simulink library "TempSensor"  (Simulink 7.6)
settings: Solver=ode1  StartTime=0.0  StopTime=Inf  FixedStep=0.001  RelTol=1e-3
PostLoadFcn:
  | , if any(exist('dsrtsu_mdlpostloadfcn', 'file') == [2, 3, 6]), try dsrtsu_mdlpostloadfcn('Execute', bdroot); catch fprintf('Error in PostLoadFcn (dsrtsu_mdlpostloadfcn) for model "%s":\n %s\n', bdroot, lasterr); end, end,
libraries: rti1401lib_dac_type1 x1
settings Model: DSRTSU_INTERNAL_RTI_VER=370  DSRTSU_INTERNAL_RTI_TYPE=rti1401  Creator=ses  LastModifiedBy=ses

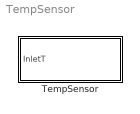
== system TempSensor ==
  TempSensor : Subsystem  mask{R0=200, TSnsrVect=[1 3.8285e-3 -5.85e-7], PuUpR=1000, PuUpU=5, CalBias=-0.006}
      mask prompts: R0 "Nominal Resistance [Ohm]"; TSnsrVect "Sensor Characteristic Vector"; PuUpR "Pull-up Resistance [Ohm]"; PuUpU "Pull-up Voltage [V]"; CalBias "Calibration Bias"

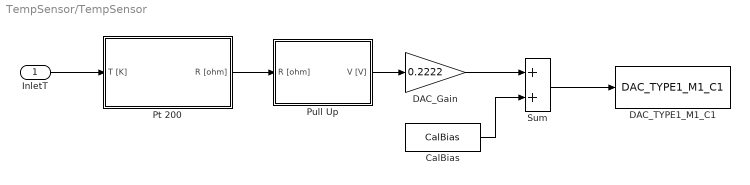
== system TempSensor/TempSensor ==
  InletT : Inport
  CalBias : Constant  Value=CalBias
  DAC_Gain : Gain  Gain=0.2222
  DAC_TYPE1_M1_C1 : rti1401lib_dac_type1/DAC_TYPE1_M1_C1  SystemSampleTime=-1  ModuleNo=1  ChannelNo=1  VoltageInitValue=0  VoltageTermMode=off  VoltageTermValue=0  Reserved1=[]  Reserved2=[]  Reserved3=[]  Reserved4=[]  DSProperties=struct('RTI',struct('Version',uint32(1),'BlockType',struct('isSLSource',uint8(0),'isSLSink',uint8(1),'isHWSource',uint8(0),'isHWSink',uint8(1),'isSetup',uint8(0),'isInline',uint8(0),'isNonInline',uint8(1),'isInterrupt',uint8(0),'isChannelwise',uint8(1)),'IOBoardType','DS1401STANDARD','UnitType','DAC','Identifier','DAC_TYPE1','DialogType','SL','BlockSet','NONE','SlaveProcessor','NONE'))  RTIBlockInterface=struct('InputPortsActive',1,'BlockDisplay',{{'DAC','center'}},'IconTransparency','off','InitLevel',1,'BlockName',struct('Token',{{'DAC_TYPE1_M','_C'}},'BlockParam',{{'ModuleNo','ChannelNo'}}),'MaskDescription',['Channel-wise write access to the 8 DAC channels'])  RTIBlockParameters=struct('ModuleNo',{{1,'ON',[1 16]}},'ChannelNo',{{1,'ON',[1 8]}},'VoltageInitValue',{{0,'ON',[0 4.5]}},'VoltageTermMode',{{logical(0),'ON',[0 1]}},'VoltageTermValue',{{0,'VoltageTermMode',[0 4.5]}})  RTISFcnParameters=struct('ModuleNo','double','ChannelNo','double','VoltageInitValue','double','VoltageTermMode','double','VoltageTermValue','double')  RTIBlockParaDefault=struct('ModuleNo',1,'ChannelNo',1,'VoltageInitValue',0,'VoltageTermMode',0,'VoltageTermValue',0)
  Pt 200 : Subsystem
  Pull Up : Subsystem
  Sum : Sum
  wires:
  InletT/1 -> Pt 200/1(T [K])
  Pt 200/1(R [ohm]) -> Pull Up/1(R [ohm])
  Pull Up/1(V [V]) -> DAC_Gain/1
  DAC_Gain/1 -> Sum/1
  Sum/1 -> DAC_TYPE1_M1_C1/1
  CalBias/1 -> Sum/2

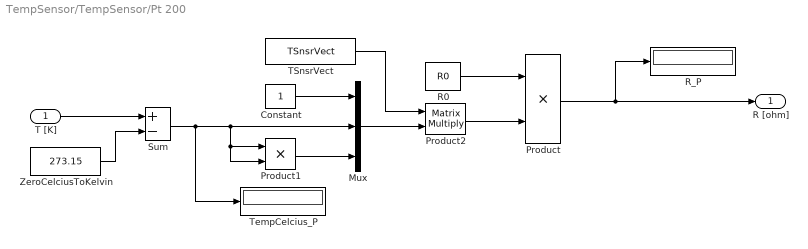
== system TempSensor/TempSensor/Pt 200 ==
  T [K] : Inport
  Constant : Constant
  Mux : Mux  Inputs=3
  Product : Product  RndMeth=Zero
  Product1 : Product  RndMeth=Zero
  Product2 : Product  Multiplication=Matrix(*)  RndMeth=Zero
  R0 : Constant  Value=R0
  R_P : Display
  Sum : Sum  Inputs=+-
  TSnsrVect : Constant  Value=TSnsrVect  VectorParams1D=off
  TempCelcius_P : Display
  ZeroCelciusToKelvin : Constant  Value=273.15
  R [ohm] : Outport
  wires:
  Constant/1 -> Mux/1
  Product1/1 -> Mux/3
  Mux/1 -> Product2/2
  TSnsrVect/1 -> Product2/1
  Product2/1 -> Product/2
  R0/1 -> Product/1
  Product/1 -> R [ohm]/1, R_P/1
  Sum/1 -> Mux/2, Product1/1, Product1/2, TempCelcius_P/1
  T [K]/1 -> Sum/1
  ZeroCelciusToKelvin/1 -> Sum/2

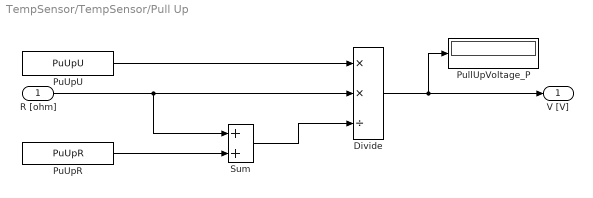
== system TempSensor/TempSensor/Pull Up ==
  R [ohm] : Inport
  Divide : Product  Inputs=**/
  PuUpR : Constant  Value=PuUpR
  PuUpU : Constant  Value=PuUpU
  PullUpVoltage_P : Display
  Sum : Sum
  V [V] : Outport
  wires:
  PuUpU/1 -> Divide/1
  Sum/1 -> Divide/3
  PuUpR/1 -> Sum/2
  R [ohm]/1 -> Divide/2, Sum/1
  Divide/1 -> V [V]/1, PullUpVoltage_P/1
